simulink model "Room_model_with_subsystem_2015a"  (R2015a)
settings: Solver=ode45  StartTime=0.0  StopTime=200  RelTol=1e-3
InitFcn:
  | server = Sim_server(10000);
StopFcn:
  | server.stop
undefined symbols (not defined in the file): Cth, Rth, x1, x2, x3, y1, y2, y3
libraries: simulink x1
settings Model: CovModelRefEnable=off  Creator=e0154145  LastModifiedBy=accma
settings DataIOCC: LimitDataPoints=off  SaveFormat=Dataset
settings HardwareCC: ProdBitPerPointer=64  ProdLargestAtomicFloat=Float  ProdIntDivRoundTo=Zero  ProdEndianess=LittleEndian  ProdHWDeviceType=Specified
settings ModelReferenceCC: PropagateSignalLabelsOutOfModel=on

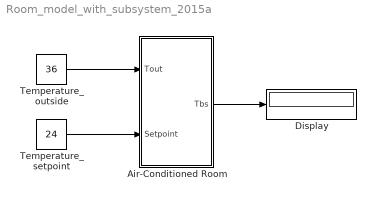
== system Room_model_with_subsystem_2015a ==
  Air-Conditioned Room : Subsystem
  Display : Display
  Temperature_outside : Constant  Value=36
  Temperature_setpoint : Constant  Value=24
  wires:
  Temperature_outside/1 -> Air-Conditioned Room/1(Tout)
  Temperature_setpoint/1 -> Air-Conditioned Room/2(Setpoint)
  Air-Conditioned Room/1(Tbs) -> Display/1

== system Room_model_with_subsystem_2015a/Air-Conditioned Room ==
  Tout : Inport
  Setpoint : Inport  Port=2
  Control : Subsystem
  Room : Subsystem
  Tbs : Outport
  wires:
  Setpoint/1 -> Control/2(Setpoint)
  Room/1(Tbs) -> Tbs/1, Control/1("Tbs ")
  Control/1("Qhvac ") -> Room/2(Qhvac)
  Tout/1 -> Room/1(Tout)

== system Room_model_with_subsystem_2015a/Air-Conditioned Room/Control ==
  "Tbs " : Inport
  Setpoint : Inport  Port=2
  PID Controller1 : simulink/Continuous/PID Controller  Controller=PID  TimeDomain=Continuous-time  SampleTime=-1  IntegratorMethod=Forward Euler  FilterMethod=Forward Euler  Form=Parallel  UseFilter=on  ControllerParametersSource=internal  P=-48.5287946828106  I=-345.034799736216  D=-0.161133654003053  N=216.924955724861  InitialConditionSource=internal  InitialConditionForIntegrator=0  InitialConditionForFilter=0  ExternalReset=none  LimitOutput=on  UpperSaturationLimit=20  LowerSaturationLimit=16  LinearizeAsGain=on  AntiWindupMode=back-calculation  Kb=1  TrackingMode=off  Kt=1  PParamMin=[]  PParamMax=[]  IParamMin=[]  IParamMax=[]  DParamMin=[]  DParamMax=[]  NParamMin=[]  NParamMax=[]  KbParamMin=[]  KbParamMax=[]  KtParamMin=[]  KtParamMax=[]  POutMin=[]  POutMax=[]  IOutMin=[]  IOutMax=[]  DOutMin=[]  DOutMax=[]  NOutMin=[]  NOutMax=[]  KbOutMin=[]  KbOutMax=[]  KtOutMin=[]  KtOutMax=[]  IntegratorOutMin=[]  IntegratorOutMax=[]  FilterOutMin=[]  FilterOutMax=[]  SumOutMin=[]  SumOutMax=[]  SumI1OutMin=[]  SumI1OutMax=[]  SumI2OutMin=[]  SumI2OutMax=[]  SumI3OutMin=[]  SumI3OutMax=[]  SumDOutMin=[]  SumDOutMax=[]  SaturationOutMin=[]  SaturationOutMax=[]  IntegratorContinuousStateAttributes=''  IntegratorStateMustResolveToSignalObject=off  IntegratorRTWStateStorageClass=Auto  FilterContinuousStateAttributes=''  FilterStateMustResolveToSignalObject=off  FilterRTWStateStorageClass=Auto  DifferentiatorICPrevScaledInput=0  DifferentiatorOutMin=[]  DifferentiatorOutMax=[]
  Sum : Sum  Inputs=+-
  "Qhvac " : Outport
  wires:
  Setpoint/1 -> Sum/1
  PID Controller1/1 -> "Qhvac "/1
  Sum/1 -> PID Controller1/1
  "Tbs "/1 -> Sum/2

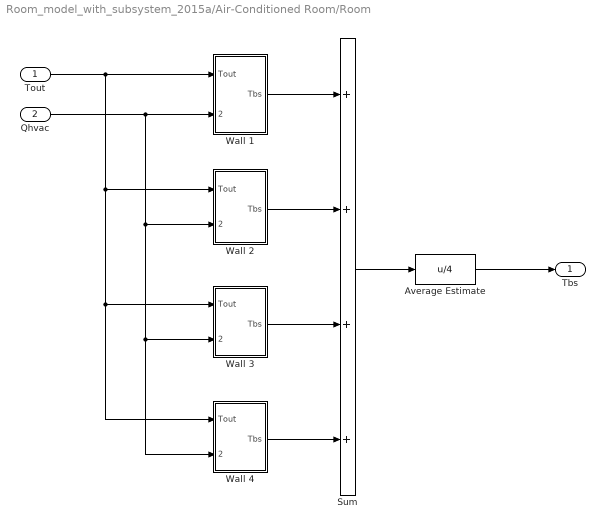
== system Room_model_with_subsystem_2015a/Air-Conditioned Room/Room ==
  Tout : Inport
  Qhvac : Inport  Port=2
  Average Estimate : Fcn  Expr=u/4
  Sum : Sum  Inputs=++++
  "Wall 1 " : Subsystem
  Wall 2 : Subsystem
  Wall 3 : Subsystem
  Wall 4 : Subsystem
  Tbs : Outport
  wires:
  Tout/1 -> Wall 4/1(Tout), Wall 3/1(Tout), Wall 2/1(Tout), "Wall 1 "/1(Tout)
  Wall 4/1("Tbs ") -> Sum/4
  Average Estimate/1 -> Tbs/1
  Wall 3/1("Tbs ") -> Sum/3
  "Wall 1 "/1("Tbs ") -> Sum/1
  Sum/1 -> Average Estimate/1
  Qhvac/1 -> Wall 4/2(Qhvac), Wall 3/2(Qhvac), Wall 2/2(Qhvac), "Wall 1 "/2(Qhvac)
  Wall 2/1("Tbs ") -> Sum/2

== system Room_model_with_subsystem_2015a/Air-Conditioned Room/Room/Wall 1  ==
  Tout : Inport
  Qhvac : Inport  Port=2
  Subsystem : Subsystem
  Subsystem1 : Subsystem
  Subsystem2 : Subsystem
  "Tbs " : Outport
  wires:
  Tout/1 -> Subsystem/1(Tout)
  Subsystem2/1("Tbs ") -> Subsystem1/3(Tbs), "Tbs "/1
  Subsystem/1(T1) -> Subsystem1/1("T1 ")
  Qhvac/1 -> Subsystem1/2(Qhvac), Subsystem2/1("Qhvac ")
  Subsystem1/1("T2 ") -> Subsystem2/2("T2 "), Subsystem/2(T2)

== system Room_model_with_subsystem_2015a/Air-Conditioned Room/Room/Wall 2 ==
  Tout : Inport
  Qhvac : Inport  Port=2
  Subsystem : Subsystem
  Subsystem1 : Subsystem
  Subsystem2 : Subsystem
  "Tbs " : Outport
  wires:
  Tout/1 -> Subsystem/1(Tout)
  Subsystem2/1("Tbs ") -> Subsystem1/3(Tbs), "Tbs "/1
  Subsystem/1(T1) -> Subsystem1/1("T1 ")
  Qhvac/1 -> Subsystem1/2(Qhvac), Subsystem2/1("Qhvac ")
  Subsystem1/1("T2 ") -> Subsystem2/2("T2 "), Subsystem/2(T2)

== system Room_model_with_subsystem_2015a/Air-Conditioned Room/Room/Wall 3 ==
  Tout : Inport
  Qhvac : Inport  Port=2
  Subsystem : Subsystem
  Subsystem1 : Subsystem
  Subsystem2 : Subsystem
  "Tbs " : Outport
  wires:
  Tout/1 -> Subsystem/1(Tout)
  Subsystem2/1("Tbs ") -> Subsystem1/3(Tbs), "Tbs "/1
  Subsystem/1(T1) -> Subsystem1/1("T1 ")
  Qhvac/1 -> Subsystem1/2(Qhvac), Subsystem2/1("Qhvac ")
  Subsystem1/1("T2 ") -> Subsystem2/2("T2 "), Subsystem/2(T2)

== system Room_model_with_subsystem_2015a/Air-Conditioned Room/Room/Wall 4 ==
  Tout : Inport
  Qhvac : Inport  Port=2
  Subsystem : Subsystem
  Subsystem1 : Subsystem
  Subsystem2 : Subsystem
  "Tbs " : Outport
  wires:
  Tout/1 -> Subsystem/1(Tout)
  Subsystem2/1("Tbs ") -> Subsystem1/3(Tbs), "Tbs "/1
  Subsystem/1(T1) -> Subsystem1/1("T1 ")
  Qhvac/1 -> Subsystem1/2(Qhvac), Subsystem2/1("Qhvac ")
  Subsystem1/1("T2 ") -> Subsystem2/2("T2 "), Subsystem/2(T2)

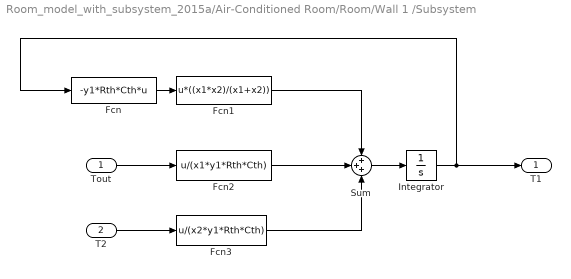
== system Room_model_with_subsystem_2015a/Air-Conditioned Room/Room/Wall 1 /Subsystem ==
  Tout : Inport
  T2 : Inport  Port=2
  Fcn : Fcn  Expr=-y1*Rth*Cth*u
  Fcn1 : Fcn  Expr=u*((x1*x2)/(x1+x2))
  Fcn2 : Fcn  Expr=u/(x1*y1*Rth*Cth)
  Fcn3 : Fcn  Expr=u/(x2*y1*Rth*Cth)
  Integrator : Integrator
  Sum : Sum  Inputs=3
  T1 : Outport
  wires:
  T2/1 -> Fcn3/1
  Fcn3/1 -> Sum/3
  Sum/1 -> Integrator/1
  Fcn2/1 -> Sum/2
  Fcn1/1 -> Sum/1
  Integrator/1 -> T1/1, Fcn/1
  Fcn/1 -> Fcn1/1
  Tout/1 -> Fcn2/1

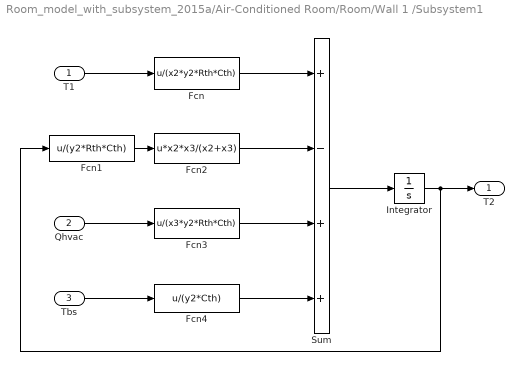
== system Room_model_with_subsystem_2015a/Air-Conditioned Room/Room/Wall 1 /Subsystem1 ==
  "T1 " : Inport
  Qhvac : Inport  Port=2
  Tbs : Inport  Port=3
  Fcn : Fcn  Expr=u/(x2*y2*Rth*Cth)
  Fcn1 : Fcn  Expr=u/(y2*Rth*Cth)
  Fcn2 : Fcn  Expr=u*x2*x3/(x2+x3)
  Fcn3 : Fcn  Expr=u/(x3*y2*Rth*Cth)
  Fcn4 : Fcn  Expr=u/(y2*Cth)
  Integrator : Integrator
  Sum : Sum  Inputs=+-++  RndMeth=Round
  "T2 " : Outport
  wires:
  Fcn1/1 -> Fcn2/1
  Integrator/1 -> "T2 "/1, Fcn1/1
  Sum/1 -> Integrator/1
  "T1 "/1 -> Fcn/1
  Qhvac/1 -> Fcn3/1
  Fcn2/1 -> Sum/2
  Tbs/1 -> Fcn4/1
  Fcn4/1 -> Sum/4
  Fcn3/1 -> Sum/3
  Fcn/1 -> Sum/1

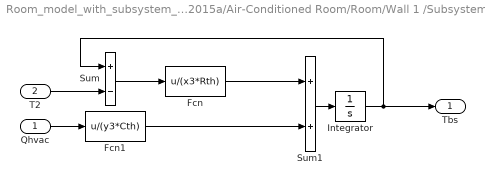
== system Room_model_with_subsystem_2015a/Air-Conditioned Room/Room/Wall 1 /Subsystem2 ==
  "Qhvac " : Inport
  "T2 " : Inport  Port=2
  Fcn : Fcn  Expr=u/(x3*Rth)
  Fcn1 : Fcn  Expr=u/(y3*Cth)
  Integrator : Integrator
  Sum : Sum  Inputs=+-
  Sum1 : Sum
  "Tbs " : Outport
  wires:
  Sum1/1 -> Integrator/1
  Fcn/1 -> Sum1/1
  Fcn1/1 -> Sum1/2
  Sum/1 -> Fcn/1
  "Qhvac "/1 -> Fcn1/1
  Integrator/1 -> "Tbs "/1, Sum/1
  "T2 "/1 -> Sum/2

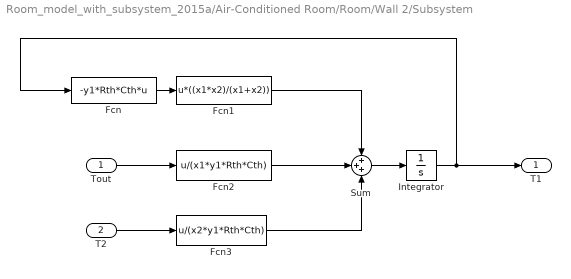
== system Room_model_with_subsystem_2015a/Air-Conditioned Room/Room/Wall 2/Subsystem ==
  Tout : Inport
  T2 : Inport  Port=2
  Fcn : Fcn  Expr=-y1*Rth*Cth*u
  Fcn1 : Fcn  Expr=u*((x1*x2)/(x1+x2))
  Fcn2 : Fcn  Expr=u/(x1*y1*Rth*Cth)
  Fcn3 : Fcn  Expr=u/(x2*y1*Rth*Cth)
  Integrator : Integrator
  Sum : Sum  Inputs=3
  T1 : Outport
  wires:
  T2/1 -> Fcn3/1
  Fcn3/1 -> Sum/3
  Sum/1 -> Integrator/1
  Fcn2/1 -> Sum/2
  Fcn1/1 -> Sum/1
  Integrator/1 -> T1/1, Fcn/1
  Fcn/1 -> Fcn1/1
  Tout/1 -> Fcn2/1

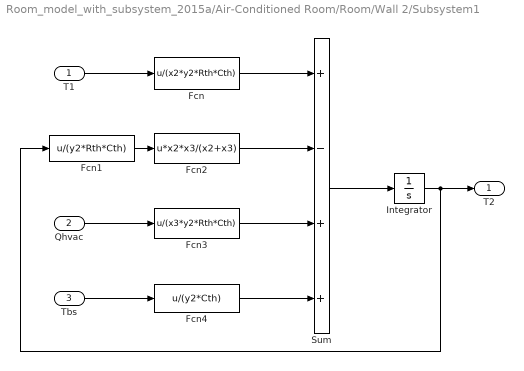
== system Room_model_with_subsystem_2015a/Air-Conditioned Room/Room/Wall 2/Subsystem1 ==
  "T1 " : Inport
  Qhvac : Inport  Port=2
  Tbs : Inport  Port=3
  Fcn : Fcn  Expr=u/(x2*y2*Rth*Cth)
  Fcn1 : Fcn  Expr=u/(y2*Rth*Cth)
  Fcn2 : Fcn  Expr=u*x2*x3/(x2+x3)
  Fcn3 : Fcn  Expr=u/(x3*y2*Rth*Cth)
  Fcn4 : Fcn  Expr=u/(y2*Cth)
  Integrator : Integrator
  Sum : Sum  Inputs=+-++  RndMeth=Round
  "T2 " : Outport
  wires:
  Fcn1/1 -> Fcn2/1
  Integrator/1 -> "T2 "/1, Fcn1/1
  Sum/1 -> Integrator/1
  "T1 "/1 -> Fcn/1
  Qhvac/1 -> Fcn3/1
  Fcn2/1 -> Sum/2
  Tbs/1 -> Fcn4/1
  Fcn4/1 -> Sum/4
  Fcn3/1 -> Sum/3
  Fcn/1 -> Sum/1

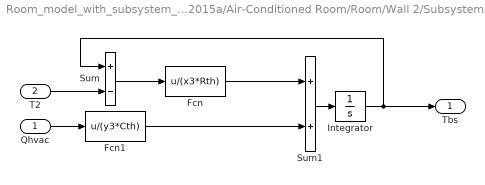
== system Room_model_with_subsystem_2015a/Air-Conditioned Room/Room/Wall 2/Subsystem2 ==
  "Qhvac " : Inport
  "T2 " : Inport  Port=2
  Fcn : Fcn  Expr=u/(x3*Rth)
  Fcn1 : Fcn  Expr=u/(y3*Cth)
  Integrator : Integrator
  Sum : Sum  Inputs=+-
  Sum1 : Sum
  "Tbs " : Outport
  wires:
  Sum1/1 -> Integrator/1
  Fcn/1 -> Sum1/1
  Fcn1/1 -> Sum1/2
  Sum/1 -> Fcn/1
  "Qhvac "/1 -> Fcn1/1
  Integrator/1 -> "Tbs "/1, Sum/1
  "T2 "/1 -> Sum/2

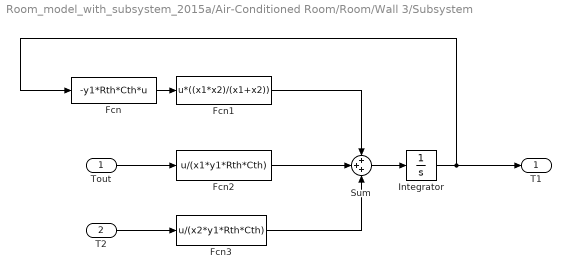
== system Room_model_with_subsystem_2015a/Air-Conditioned Room/Room/Wall 3/Subsystem ==
  Tout : Inport
  T2 : Inport  Port=2
  Fcn : Fcn  Expr=-y1*Rth*Cth*u
  Fcn1 : Fcn  Expr=u*((x1*x2)/(x1+x2))
  Fcn2 : Fcn  Expr=u/(x1*y1*Rth*Cth)
  Fcn3 : Fcn  Expr=u/(x2*y1*Rth*Cth)
  Integrator : Integrator
  Sum : Sum  Inputs=3
  T1 : Outport
  wires:
  T2/1 -> Fcn3/1
  Fcn3/1 -> Sum/3
  Sum/1 -> Integrator/1
  Fcn2/1 -> Sum/2
  Fcn1/1 -> Sum/1
  Integrator/1 -> T1/1, Fcn/1
  Fcn/1 -> Fcn1/1
  Tout/1 -> Fcn2/1

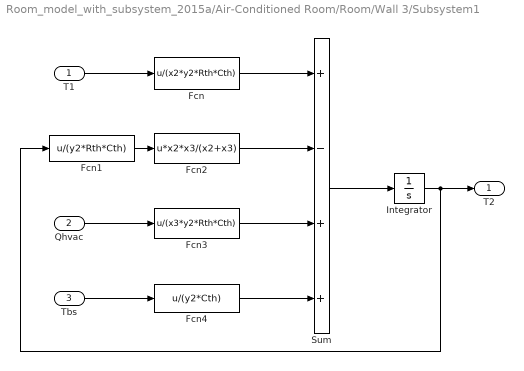
== system Room_model_with_subsystem_2015a/Air-Conditioned Room/Room/Wall 3/Subsystem1 ==
  "T1 " : Inport
  Qhvac : Inport  Port=2
  Tbs : Inport  Port=3
  Fcn : Fcn  Expr=u/(x2*y2*Rth*Cth)
  Fcn1 : Fcn  Expr=u/(y2*Rth*Cth)
  Fcn2 : Fcn  Expr=u*x2*x3/(x2+x3)
  Fcn3 : Fcn  Expr=u/(x3*y2*Rth*Cth)
  Fcn4 : Fcn  Expr=u/(y2*Cth)
  Integrator : Integrator
  Sum : Sum  Inputs=+-++  RndMeth=Round
  "T2 " : Outport
  wires:
  Fcn1/1 -> Fcn2/1
  Integrator/1 -> "T2 "/1, Fcn1/1
  Sum/1 -> Integrator/1
  "T1 "/1 -> Fcn/1
  Qhvac/1 -> Fcn3/1
  Fcn2/1 -> Sum/2
  Tbs/1 -> Fcn4/1
  Fcn4/1 -> Sum/4
  Fcn3/1 -> Sum/3
  Fcn/1 -> Sum/1

== system Room_model_with_subsystem_2015a/Air-Conditioned Room/Room/Wall 3/Subsystem2 ==
  "Qhvac " : Inport
  "T2 " : Inport  Port=2
  Fcn : Fcn  Expr=u/(x3*Rth)
  Fcn1 : Fcn  Expr=u/(y3*Cth)
  Integrator : Integrator
  Sum : Sum  Inputs=+-
  Sum1 : Sum
  "Tbs " : Outport
  wires:
  Sum1/1 -> Integrator/1
  Fcn/1 -> Sum1/1
  Fcn1/1 -> Sum1/2
  Sum/1 -> Fcn/1
  "Qhvac "/1 -> Fcn1/1
  Integrator/1 -> "Tbs "/1, Sum/1
  "T2 "/1 -> Sum/2

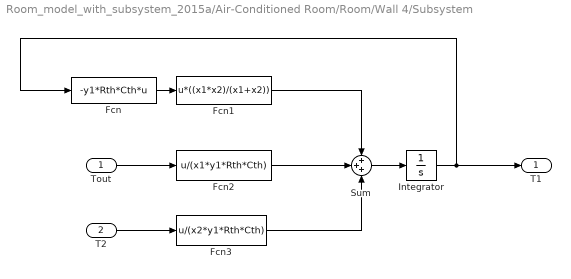
== system Room_model_with_subsystem_2015a/Air-Conditioned Room/Room/Wall 4/Subsystem ==
  Tout : Inport
  T2 : Inport  Port=2
  Fcn : Fcn  Expr=-y1*Rth*Cth*u
  Fcn1 : Fcn  Expr=u*((x1*x2)/(x1+x2))
  Fcn2 : Fcn  Expr=u/(x1*y1*Rth*Cth)
  Fcn3 : Fcn  Expr=u/(x2*y1*Rth*Cth)
  Integrator : Integrator
  Sum : Sum  Inputs=3
  T1 : Outport
  wires:
  T2/1 -> Fcn3/1
  Fcn3/1 -> Sum/3
  Sum/1 -> Integrator/1
  Fcn2/1 -> Sum/2
  Fcn1/1 -> Sum/1
  Integrator/1 -> T1/1, Fcn/1
  Fcn/1 -> Fcn1/1
  Tout/1 -> Fcn2/1

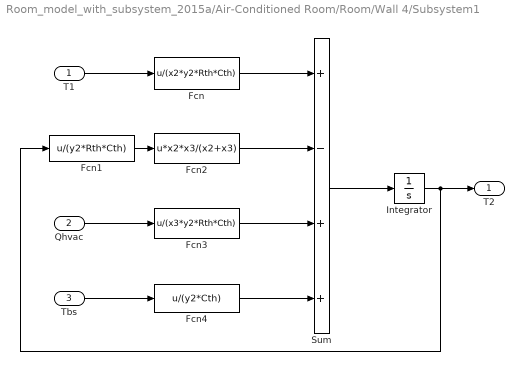
== system Room_model_with_subsystem_2015a/Air-Conditioned Room/Room/Wall 4/Subsystem1 ==
  "T1 " : Inport
  Qhvac : Inport  Port=2
  Tbs : Inport  Port=3
  Fcn : Fcn  Expr=u/(x2*y2*Rth*Cth)
  Fcn1 : Fcn  Expr=u/(y2*Rth*Cth)
  Fcn2 : Fcn  Expr=u*x2*x3/(x2+x3)
  Fcn3 : Fcn  Expr=u/(x3*y2*Rth*Cth)
  Fcn4 : Fcn  Expr=u/(y2*Cth)
  Integrator : Integrator
  Sum : Sum  Inputs=+-++  RndMeth=Round
  "T2 " : Outport
  wires:
  Fcn1/1 -> Fcn2/1
  Integrator/1 -> "T2 "/1, Fcn1/1
  Sum/1 -> Integrator/1
  "T1 "/1 -> Fcn/1
  Qhvac/1 -> Fcn3/1
  Fcn2/1 -> Sum/2
  Tbs/1 -> Fcn4/1
  Fcn4/1 -> Sum/4
  Fcn3/1 -> Sum/3
  Fcn/1 -> Sum/1

== system Room_model_with_subsystem_2015a/Air-Conditioned Room/Room/Wall 4/Subsystem2 ==
  "Qhvac " : Inport
  "T2 " : Inport  Port=2
  Fcn : Fcn  Expr=u/(x3*Rth)
  Fcn1 : Fcn  Expr=u/(y3*Cth)
  Integrator : Integrator
  Sum : Sum  Inputs=+-
  Sum1 : Sum
  "Tbs " : Outport
  wires:
  Sum1/1 -> Integrator/1
  Fcn/1 -> Sum1/1
  Fcn1/1 -> Sum1/2
  Sum/1 -> Fcn/1
  "Qhvac "/1 -> Fcn1/1
  Integrator/1 -> "Tbs "/1, Sum/1
  "T2 "/1 -> Sum/2
